simulink subsystem "Unity_Visualizer"  (R2023b)
settings: Solver=VariableStepAuto  StartTime=0.0  StopTime=10.0  RelTol=1e-3
libraries: simulink_extras x7, dspnetwork x1
settings Model: Creator=cyber  LastModifiedBy=cyber

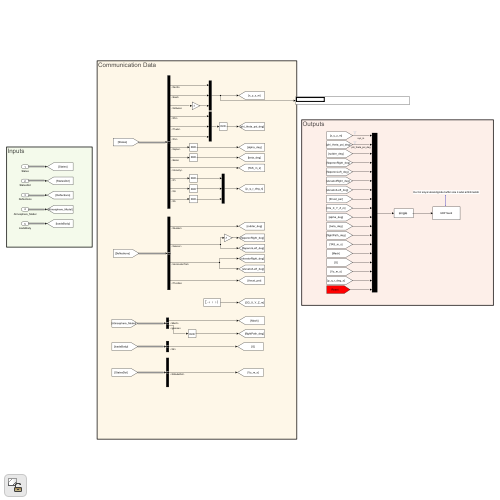
[thumbnail: Simulink's stored preview of the top-level diagram]
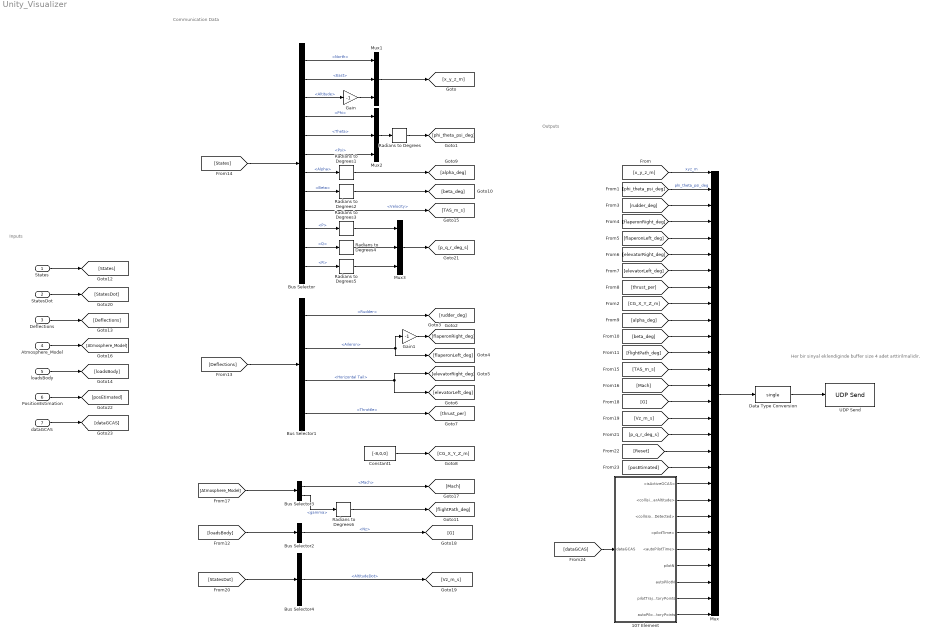
== system Unity_Visualizer ==
  note: Her bir sinyal eklendiginde buffer size 4 adet arttirilmalidir.
  note: Inputs
  note: Outputs
  note: Communication Data
  States : Inport
  StatesDot : Inport  Port=2
  Deflections : Inport  Port=3
  Atmosphere_Model : Inport  Port=4
  loadsBody : Inport  Port=5
  PositionEstimation : Inport  Port=6
  dataGCAS : Inport  Port=7
  107 Element : Subsystem
  Bus Selector : BusSelector  OutputSignals=North,East,Altitude,Phi,Theta,Psi,Alpha,Beta,Velocity,P,Q,R
  Bus Selector1 : BusSelector  OutputSignals=Rudder,Aileron,Horizontal Tail,Throttle
  Bus Selector2 : BusSelector  OutputSignals=Nz
  Bus Selector3 : BusSelector  OutputSignals=Mach,gamma
  Bus Selector4 : BusSelector  OutputSignals=AltitudeDot
  Constant1 : Constant  Value=[-8,0,0]
  Data Type Conversion : DataTypeConversion  OutDataTypeStr=single  SaturateOnIntegerOverflow=off  RndMeth=Floor
  Gain : Gain  Gain=-1
  Gain1 : Gain  Gain=-1
  Mux : Mux  Inputs=28
  Mux1 : Mux  Inputs=3
  Mux2 : Mux  Inputs=3
  Mux3 : Mux  Inputs=3
  Radians to Degrees{,1..6} (7 alike) : simulink_extras/Transformations/Radians to Degrees
  UDP Send : dspnetwork/UDP Send  remoteURL=stateSenderIP  remotePort=stateSenderPort  localURL='0.0.0.0'  localPortSource=Automatically determine  localPort=-1  sendBufferSize=29*4 + 107*4  sampletime=-1  blockPlatform=[]  separateLengthPort=0
  wires:
  [flaperonRight_deg] -> Mux/4
  [CG_X_Y_Z_m] -> Mux/9
  [thrust_per] -> Mux/8
  [phi_theta_psi_deg] -> Mux/2  "phi_theta_psi_deg"
  [elevatorRight_deg] -> Mux/6
  [elevatorLeft_deg] -> Mux/7
  Mux/1 -> Data Type Conversion/1
  [alpha_deg] -> Mux/10
  [rudder_deg] -> Mux/3
  [flightPath_deg] -> Mux/12
  Data Type Conversion/1 -> UDP Send/1
  [flaperonLeft_deg] -> Mux/5
  [beta_deg] -> Mux/11
  [x_y_z_m] -> Mux/1  "xyz_m"
  [States] -> Bus Selector/1
  Bus Selector/1 -> Mux1/1  "<North>"
  Bus Selector/2 -> Mux1/2  "<East>"
  Bus Selector/3 -> Gain/1  "<Altitude>"
  Gain/1 -> Mux1/3
  Mux1/1 -> [x_y_z_m]
  Bus Selector/4 -> Mux2/1  "<Phi>"
  Bus Selector/5 -> Mux2/2  "<Theta>"
  Bus Selector/6 -> Mux2/3  "<Psi>"
  Mux2/1 -> Radians to Degrees/1
  Radians to Degrees/1 -> [phi_theta_psi_deg]
  [Deflections] -> Bus Selector1/1
  Bus Selector1/1 -> [rudder_deg]  "<Rudder>"
  Bus Selector1/2 -> Gain1/1, [flaperonLeft_deg]  "<Aileron>"
  Bus Selector1/3 -> [elevatorLeft_deg], [elevatorRight_deg]  "<Horizontal Tail>"
  Bus Selector1/4 -> [thrust_per]  "<Throttle>"
  Gain1/1 -> [flaperonRight_deg]
  Bus Selector/7 -> Radians to Degrees1/1  "<Alpha>"
  Bus Selector/8 -> Radians to Degrees2/1  "<Beta>"
  Radians to Degrees1/1 -> [alpha_deg]
  Radians to Degrees2/1 -> [beta_deg]
  States/1 -> [States]
  Deflections/1 -> [Deflections]
  Bus Selector/9 -> [TAS_m_s]  "<Velocity>"
  [TAS_m_s] -> Mux/13
  Atmosphere_Model/1 -> [Atmosphere_Model]
  [Atmosphere_Model] -> Bus Selector3/1
  Bus Selector3/1 -> [Mach]  "<Mach>"
  [Mach] -> Mux/14
  [Vz_m_s] -> Mux/16
  [G] -> Mux/15
  [loadsBody] -> Bus Selector2/1
  StatesDot/1 -> [StatesDot]
  [StatesDot] -> Bus Selector4/1
  Bus Selector4/1 -> [Vz_m_s]  "<AltitudeDot>"
  Bus Selector/12 -> Radians to Degrees5/1  "<R>"
  Bus Selector/11 -> Radians to Degrees4/1  "<Q>"
  Bus Selector/10 -> Radians to Degrees3/1  "<P>"
  Mux3/1 -> [p_q_r_deg_s]
  [p_q_r_deg_s] -> Mux/17
  Constant1/1 -> [CG_X_Y_Z_m]
  Radians to Degrees3/1 -> Mux3/1
  Radians to Degrees4/1 -> Mux3/2
  Radians to Degrees5/1 -> Mux3/3
  Radians to Degrees6/1 -> [flightPath_deg]
  Bus Selector3/2 -> Radians to Degrees6/1  "<gamma>"
  loadsBody/1 -> [loadsBody]
  Bus Selector2/1 -> [G]  "<Nz>"
  [Reset] -> Mux/18
  PositionEstimation/1 -> [posEtimated]
  [posEtimated] -> Mux/19
  dataGCAS/1 -> [dataGCAS]
  [dataGCAS] -> 107 Element/1(dataGCAS)
  107 Element/4(<pilotTime>) -> Mux/23
  107 Element/5(<autoPilotTime>) -> Mux/24
  107 Element/3(<collisionDetected>) -> Mux/22
  107 Element/6(pilotN) -> Mux/25
  107 Element/2(<collisionClearAltitude>) -> Mux/21
  107 Element/7(autoPilotN) -> Mux/26
  107 Element/1(<isActiveGCAS>) -> Mux/20
  107 Element/8(pilotTrajectoryPoints) -> Mux/27
  107 Element/9(autoPilotTrajectoryPoints) -> Mux/28

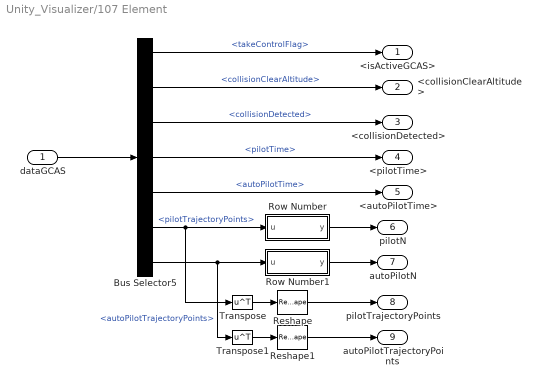
== system Unity_Visualizer/107 Element ==
  dataGCAS : Inport
  Bus Selector5 : BusSelector  OutputSignals=takeControlFlag,collisionClearAltitude,collisionDetected,pilotTime,autoPilotTime,pilotTrajectoryPoints,autoPilotTrajectoryPoints
  Reshape : Reshape  OutputDimensionality=Column vector (2-D)  OutputDimensions=[81*3,1]
  Reshape1 : Reshape  OutputDimensionality=Column vector (2-D)  OutputDimensions=[81*3,1]
  Row Number : MATLAB Function  TreatAsAtomicUnit=on
  Row Number1 : MATLAB Function  TreatAsAtomicUnit=on
  Transpose : Math  Operator=transpose
  Transpose1 : Math  Operator=transpose
  <isActiveGCAS> : Outport
  <collisionClearAltitude> : Outport  Port=2
  <collisionDetected> : Outport  Port=3
  <pilotTime> : Outport  Port=4
  <autoPilotTime> : Outport  Port=5
  pilotN : Outport  Port=6
  autoPilotN : Outport  Port=7
  pilotTrajectoryPoints : Outport  Port=8
  autoPilotTrajectoryPoints : Outport  Port=9
  wires:
  Transpose1/1 -> Reshape1/1
  Transpose/1 -> Reshape/1
  Row Number1/1(y) -> autoPilotN/1
  Row Number/1(y) -> pilotN/1
  Reshape1/1 -> autoPilotTrajectoryPoints/1
  Reshape/1 -> pilotTrajectoryPoints/1
  Bus Selector5/7 -> Row Number1/1(u), Transpose1/1  "<autoPilotTrajectoryPoints>"
  Bus Selector5/3 -> <collisionDetected>/1  "<collisionDetected>"
  Bus Selector5/2 -> <collisionClearAltitude>/1  "<collisionClearAltitude>"
  Bus Selector5/5 -> <autoPilotTime>/1  "<autoPilotTime>"
  Bus Selector5/4 -> <pilotTime>/1  "<pilotTime>"
  Bus Selector5/1 -> <isActiveGCAS>/1  "<takeControlFlag>"
  Bus Selector5/6 -> Transpose/1, Row Number/1(u)  "<pilotTrajectoryPoints>"
  dataGCAS/1 -> Bus Selector5/1

== matlab function Unity_Visualizer/107 Element/Row Number1 ==
  data: u input; y output
function y = fcn(u)
[rowN,colN] = size(u);
y = rowN;

== matlab function Unity_Visualizer/107 Element/Row Number ==
  data: u input; y output
function y = fcn(u)
[rowN,colN] = size(u);
y = rowN;
